simulink model "LADRC_24aV3_0"  (R2025a)
settings: Solver=VariableStepAuto  StartTime=0  StopTime=10  FixedStep=0.001  RelTol=1e-5
model workspace (MAT data in the model file):
  Amp = 0.0011
  P = 0
values from neighbouring files (symbols this model uses):
  A1 = 3.1416e-04    (= 0.00031416)    [InitialParameter.m]    (also in pneumatic_code.m = 0.000314159265359)
  A2 = 2.6389e-04    (= 0.00026389)    [InitialParameter.m]    (also in pneumatic_code.m = 0.000263893782902)
  Ar = 0.00005026    (= 5.026e-05)    [InitialParameter.m]    (also in pneumatic_code.m = 5.02654824574e-05)
  b = 1    [InitialParameter.m]    (also in pneumatic_code.m = 0.0025)
  beta = 50    [InitialParameter.m]
  bs = 0.008    [InitialParameter.m]
  ep = 0.0024    [InitialParameter.m]    (also in pneumatic_code.m = 0.02)
  g1 = 9    [InitialParameter.m]    (also in pneumatic_code.m = 10)
  g2 = 4    [InitialParameter.m]    (also in pneumatic_code.m = 9)
  g3 = 18    [InitialParameter.m]    (also in pneumatic_code.m = 5)
  g4 = 0.32    [InitialParameter.m]    (also in pneumatic_code.m = 3)
  g5 = 3    [pneumatic_code.m]
  k1 = wc^4    (= 81450625)    [InitialParameter.m]    (also in pneumatic_code.m = 3620506.28125)
  k2 = 4*wc^3    (= 3429500)    [InitialParameter.m]    (also in pneumatic_code.m = 883050.3125)
  k3 = 6*wc^2    (= 54150)    [InitialParameter.m]    (also in pneumatic_code.m = 86151.25)
  k4 = 4*wc    (= 380)    [InitialParameter.m]    (also in pneumatic_code.m = 4202.5)
  k5 = 5*(wc)    (= 102.5)    [pneumatic_code.m]
  Ke = 50    [InitialParameter.m]
  L = 0.15    [InitialParameter.m]    (also in pneumatic_code.m)
  M = 0.1    [InitialParameter.m]    (also in pneumatic_code.m)
  Ms = 0.5    [InitialParameter.m]    (also in pneumatic_code.m)
  Pa = 101352    [InitialParameter.m]
  Rs = 13.5    [InitialParameter.m]    (also in pneumatic_code.m)
  Vinact = 1e-04    (= 0.0001)    [InitialParameter.m]    (also in pneumatic_code.m)
  wall_force = 1e12    (= 1000000000000)    [InitialParameter.m]
  WallPos = 0.1    [InitialParameter.m]
undefined symbols (not defined in the file or in its folder): sigbuilder_block
libraries: slpidlib x1, SignalEditorBlockLib x1
settings Model: Creator=ply  LastModifiedBy=pangl
settings SolverCC: ZeroCrossAlgorithm=Adaptive
settings OptimizationCC: ZeroExternalMemoryAtStartup=off  ZeroInternalMemoryAtStartup=off
settings DebuggingCC: IgnoredZcDiagnostic=none  UnderSpecifiedDimensionMsg=warning
settings RTWCC: TargetLang=C++
settings GRTTargetCC: TargetLangStandard=C++11 (ISO)  CodeInterfacePackaging=C++ class

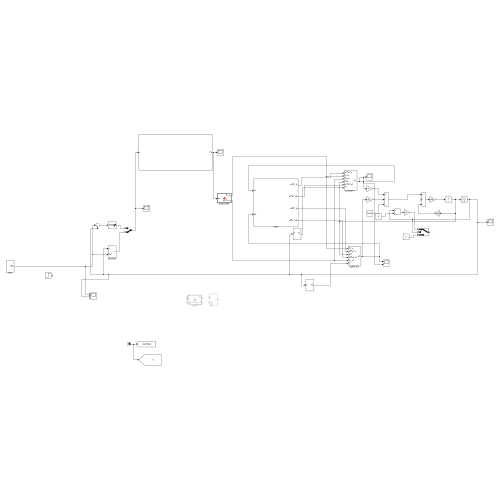
[thumbnail: Simulink's stored preview of the top-level diagram]
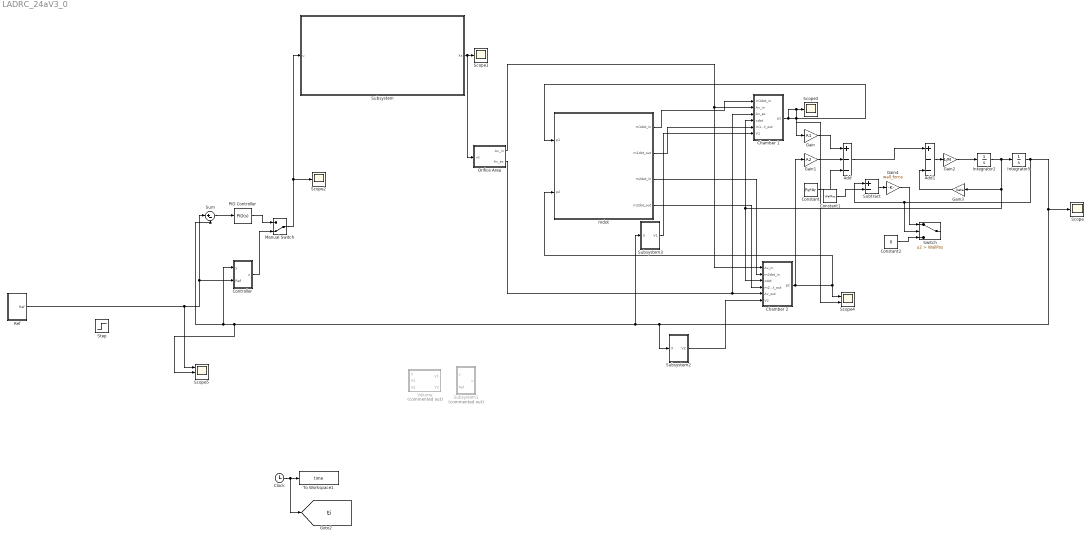
== system LADRC_24aV3_0 ==
  Add : Sum  Inputs=+--
  Add1 : Sum  Inputs=+--
  "Chamber 1 " : Subsystem
  Chamber 2 : Subsystem
  Clock : Clock
  Constant : Constant  Value=Pa*Ar
  Constant1 : Constant  Value=WallPos
  Constant2 : Constant  Value=0
  Controller : Subsystem
  Gain : Gain  Gain=A1
  Gain1 : Gain  Gain=A2
  Gain2 : Gain  Gain=1/M
  Gain3 : Gain  Gain=beta
  Gain4 : Gain  Gain=wall_force
  Integrator2 : Integrator
  Integrator5 : Integrator  InitialCondition=1e-4  LimitOutput=on  UpperSaturationLimit=0.15  LowerSaturationLimit=1e-4
  Manual Switch : ManualSwitch  CurrentSetting=0
  Orifice Area : MATLAB Function  TreatAsAtomicUnit=on
  PID Controller : slpidlib/PID Controller  Controller=PID  Form=Parallel  TimeDomain=Continuous-time  UseExternalTs=off  SampleTime=-1  IntegratorMethod=Forward Euler  FilterMethod=Forward Euler  ControllerParametersSource=internal  P=3800  I=420  UseKiTs=off  D=260  UseExternalDerivativeSource=off  N=4500  UseFilter=on  TunerSelectOption=Transfer Function Based (PID Tuner App)  InitialConditionSource=internal  InitialConditionForIntegrator=0  InitialConditionForFilter=19  DifferentiatorICPrevScaledInput=0  ExternalReset=none  TrackingMode=off  Kt=1  LimitOutput=on  SatLimitsSource=internal  UpperSaturationLimit=20  LowerSaturationLimit=-20  LinearizeAsGain=off  AntiWindupMode=clamping  Kb=2  LimitIntegrator=off  UpperIntegratorSaturationLimit=inf  LowerIntegratorSaturationLimit=-inf  POutMin=[]  POutMax=[]  IOutMin=[]  IOutMax=[]  DOutMin=[]  DOutMax=[]  NOutMin=[]  NOutMax=[]  SumOutMin=[]  SumOutMax=[]  SaturationOutMin=[]  SaturationOutMax=[]  PParamMin=[]  PParamMax=[]  IParamMin=[]  IParamMax=[]  DParamMin=[]  DParamMax=[]  NParamMin=[]  NParamMax=[]  KbParamMin=[]  KbParamMax=[]  KtParamMin=[]  KtParamMax=[]  KbOutMin=[]  KbOutMax=[]  KtOutMin=[]  KtOutMax=[]  IntegratorOutMin=[]  IntegratorOutMax=[]  FilterOutMin=[]  FilterOutMax=[]  SumI1OutMin=[]  SumI1OutMax=[]  SumI2OutMin=[]  SumI2OutMax=[]  SumI3OutMin=[]  SumI3OutMax=[]  SumI4OutMin=[]  SumI4OutMax=[]  SumDOutMin=[]  SumDOutMax=[]  DifferentiatorOutMin=[]  DifferentiatorOutMax=[]  FilterDiffOutCoefMin=[]  FilterDiffOutCoefMax=[]  ReciprocalOutMin=[]  ReciprocalOutMax=[]  SumDenOutMin=[]  SumDenOutMax=[]  SumNumOutMin=[]  SumNumOutMax=[]  DivideOutMin=[]  DivideOutMax=[]  UdiffTsProdOutMin=[]  UdiffTsProdOutMax=[]  NTsProdOutMin=[]  NTsProdOutMax=[]  UintegralTsProdOutMin=[]  UintegralTsProdOutMax=[]  UngainTsProdOutMin=[]  UngainTsProdOutMax=[]  ClampingZeroOutDataTypeStr=Inherit: Inherit via back propagation  ClampingZeroOutMin=[]  ClampingZeroOutMax=[]  FilterDenConstantOutDataTypeStr=Inherit: Inherit via back propagation  FilterDenConstantOutMin=[]  FilterDenConstantOutMax=[]  PCopyOutDataTypeStr=Inherit: Inherit via back propagation  PCopyOutMin=[]  PCopyOutMax=[]  NCopyOutDataTypeStr=Inherit: Inherit via back propagation  NCopyOutMin=[]  NCopyOutMax=[]  IntegratorContinuousStateAttributes=''  IntegratorStateMustResolveToSignalObject=off  IntegratorRTWStateStorageClass=Auto  FilterContinuousStateAttributes=''  FilterStateMustResolveToSignalObject=off  FilterRTWStateStorageClass=Auto  ParallelPVariant=InternalParameters  IdealPVariant=Disabled  IVariant=InternalParameters  DVariant=InternalParameters  IntegratorVariant=Continuous  SatVariant=Enabled  AWVariant=ContClampingParallel  PCopyVariant=Disabled  TRVariant=Disabled  FdbkBlocksVariant=Forward  IdealPFdbkVariant=Disabled  SatFdbkVariant=Disabled  DerivativeFilterVariant=ContFilter  NVariant=InternalParameters  NCopyVariant=Disabled  FilterICVariant=InternalICsFilter  IntegratorICVariant=InternalICs  ExternalResetVariant=Disabled  TRSumVariant=Passthrough  SumFdbkVariant=Disabled  SumVariant=Sum_PID  TsampFilterVariant=InternalTs  TsampNgainVariant=Passthrough  TsampIntegralVariant=Disabled_SignalSpec  ExternalSaturationOutDataTypeStr=Inherit: Same as second input  DerivativeSourceVariant=ErrorSignal  PreIntVariant=InternalPreInt
  Ref : Subsystem
  Scope{,1..3} (4 alike) : Scope
      Scope settings: ActiveDisplayYMinimum=-0.01125  ActiveDisplayYMaximum=0.10227
      Scope1 settings: ActiveDisplayYMinimum=-0.00138  ActiveDisplayYMaximum=0.00138  DataLoggingVariableName=ScopeData2
      Scope2 settings: ActiveDisplayYMinimum=-25  ActiveDisplayYMaximum=25  DataLoggingVariableName=ScopeData2
      Scope3 settings: ActiveDisplayYMinimum=39461.93859  ActiveDisplayYMaximum=658362.55266  DataLoggingVariableName=ScopeData3
  Scope4 : Scope  NumInputPorts=2
      settings: ActiveDisplayYMinimum=-74914.57533  ActiveDisplayYMaximum=775581.17798  DataLoggingVariableName=ScopeData4
  Scope5 : Scope  NumInputPorts=3
      settings: ActiveDisplayYMinimum=-0.030987006812028317  ActiveDisplayYMaximum=0.12320031519133484  DataLoggingVariableName=ScopeData7
  Step : Step  After=0.09  SampleTime=0
  Subsystem : Subsystem
  Subsystem1 : Subsystem  Commented=on
  Subsystem2 : Subsystem
  Subsystem3 : Subsystem
  Subtract : Sum  Inputs=+-
  Sum : Sum  Inputs=|+-
  Switch : Switch  Criteria=u2 > Threshold  Threshold=WallPos  SaturateOnIntegerOverflow=off  InputSameDT=off
  To Workspace1 : ToWorkspace  VariableName=time  SampleTime=-1
  Volume : MATLAB Function  Commented=on  TreatAsAtomicUnit=on
  mdot : Subsystem
  tag scope: ti=global
  wires:
  Integrator2/1 -> Gain3/1, Chamber 2/3(xdot), "Chamber 1 "/4(xdot), Integrator5/1
  "Chamber 1 "/1(p1) -> mdot/1(p1), Gain/1, Scope4/2, Scope3/1
  Orifice Area/1(Av_in) -> Chamber 2/1(Av_in), "Chamber 1 "/2(Av_in)
  Orifice Area/2(Av_ex) -> "Chamber 1 "/3(Av_ex), Chamber 2/5(Av_out)
  Chamber 2/1(p2) -> Scope4/1, mdot/2(p2), Gain1/1
  Subsystem/1(Xs) -> Orifice Area/1(xs), Scope1/1
  mdot/1(m1dot_in) -> "Chamber 1 "/1(m1dot_in)
  mdot/2(m1dot_out) -> "Chamber 1 "/5(m1dot_out)
  mdot/3(m2dot_in) -> Chamber 2/2(m2dot_in)
  mdot/4(m2dot_out) -> Chamber 2/4(m2dot_out)
  Integrator5/1 -> Switch/2, Subtract/1, Scope/1, Subsystem2/1(X), Subsystem3/1(X), Sum/2, Controller/1(y), Scope5/2
  Gain/1 -> Add/1
  Gain1/1 -> Add/2
  Constant/1 -> Add/3
  Add/1 -> Add1/1
  Gain3/1 -> Add1/3
  Add1/1 -> Gain2/1
  Constant1/1 -> Subtract/2
  Subtract/1 -> Gain4/1
  Gain4/1 -> Switch/1
  Constant2/1 -> Switch/3
  Subsystem3/1(V1) -> "Chamber 1 "/6(V1)
  Subsystem2/1(V2) -> Chamber 2/6(V2)
  Gain2/1 -> Integrator2/1
  Clock/1 -> [ti], To Workspace1/1
  PID Controller/1 -> Manual Switch/1
  Sum/1 -> PID Controller/1
  Controller/1(u) -> Manual Switch/2
  Manual Switch/1 -> Scope2/1, Subsystem/1(u)
  Ref/1(Ref) -> Sum/1, Controller/2(Ref), Scope5/1

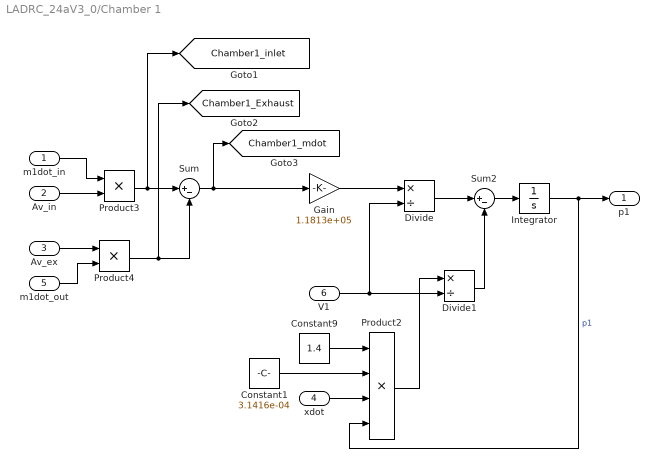
== system LADRC_24aV3_0/Chamber 1  ==
  m1dot_in : Inport
  Av_in : Inport  Port=2
  Av_ex : Inport  Port=3
  xdot : Inport  Port=4
  m1dot_out : Inport  Port=5
  V1 : Inport  Port=6
  Constant1 : Constant  Value=3.1416e-04
  Constant9 : Constant  Value=1.4
  Divide : Product  Inputs=*/
  Divide1 : Product  Inputs=*/
  Gain : Gain  Gain=1.1813e+05
  Integrator : Integrator  InitialCondition=101352  LimitOutput=on  UpperSaturationLimit=758423  LowerSaturationLimit=101352
  Product2 : Product  Inputs=4
  Product3 : Product
  Product4 : Product
  Sum : Sum  Inputs=|+-
  Sum2 : Sum  Inputs=|+-
  p1 : Outport
  tag scope: Chamber1_Exhaust=global, Chamber1_inlet=global, Chamber1_mdot=global
  wires:
  Divide/1 -> Sum2/1
  Sum/1 -> [Chamber1_mdot], Gain/1
  Gain/1 -> Divide/1
  Divide1/1 -> Sum2/2
  Constant9/1 -> Product2/1
  Product2/1 -> Divide1/1
  Integrator/1 -> p1/1, Product2/4  "p1"
  Sum2/1 -> Integrator/1
  m1dot_in/1 -> Product3/1
  xdot/1 -> Product2/3
  Product4/1 -> [Chamber1_Exhaust], Sum/2
  Av_in/1 -> Product3/2
  Product3/1 -> [Chamber1_inlet], Sum/1
  m1dot_out/1 -> Product4/2
  Av_ex/1 -> Product4/1
  Constant1/1 -> Product2/2
  V1/1 -> Divide/2, Divide1/2

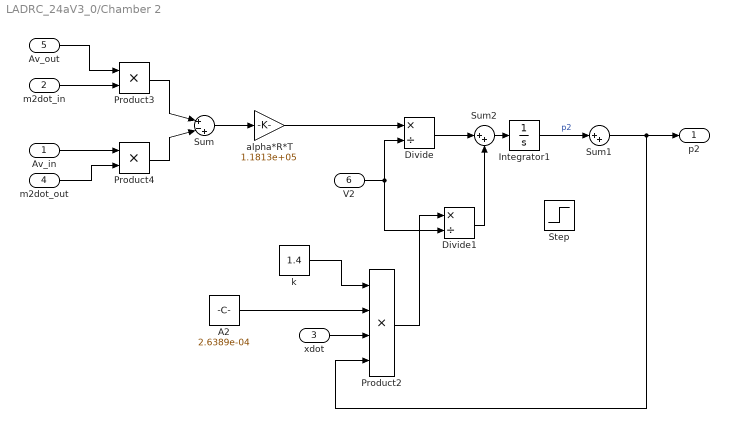
== system LADRC_24aV3_0/Chamber 2 ==
  Av_in : Inport
  m2dot_in : Inport  Port=2
  xdot : Inport  Port=3
  m2dot_out : Inport  Port=4
  Av_out : Inport  Port=5
  V2 : Inport  Port=6
  A2 : Constant  Value=2.6389e-04
  Divide : Product  Inputs=*/
  Divide1 : Product  Inputs=*/
  Integrator1 : Integrator  InitialCondition=10135  UpperSaturationLimit=75842  LowerSaturationLimit=10135
  Product2 : Product  Inputs=4
  Product3 : Product
  Product4 : Product
  Step : Step  Time=5  After=-10*10^3  SampleTime=0
  Sum : Sum  Inputs=|+-+
  Sum1 : Sum  Inputs=|++
  Sum2 : Sum  Inputs=|++
  alpha*R*T : Gain  Gain=1.1813e+05
  k : Constant  Value=1.4
  p2 : Outport
  wires:
  m2dot_out/1 -> Product4/2
  xdot/1 -> Product2/3
  Sum2/1 -> Integrator1/1
  Product2/1 -> Divide1/1
  k/1 -> Product2/1
  Divide1/1 -> Sum2/2
  A2/1 -> Product2/2
  alpha*R*T/1 -> Divide/1
  Sum/1 -> alpha*R*T/1
  Divide/1 -> Sum2/1
  Av_in/1 -> Product4/1
  m2dot_in/1 -> Product3/2
  Product3/1 -> Sum/1
  Av_out/1 -> Product3/1
  Product4/1 -> Sum/2
  V2/1 -> Divide/2, Divide1/2
  Integrator1/1 -> Sum1/1  "p2"
  Sum1/1 -> Product2/4, p2/1

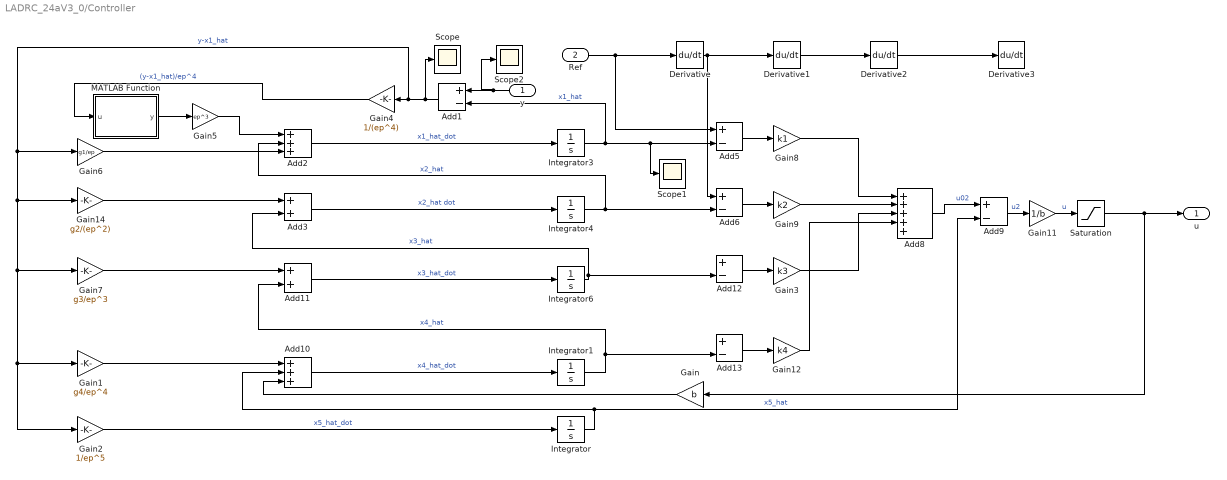
== system LADRC_24aV3_0/Controller ==
  y : Inport
  Ref : Inport  Port=2
  Add{1,5..6,9,12..13} (6 alike) : Sum  Inputs=+-
  Add10 : Sum  Inputs=+++
  Add11 : Sum
  Add2 : Sum  Inputs=+++
  Add3 : Sum
  Add8 : Sum  Inputs=+++++
  Derivative{,1..3} (4 alike) : Derivative
  Gain : Gain  Gain=b
  Gain1 : Gain  Gain=g4/ep^4
  Gain11 : Gain  Gain=1/b
  Gain12 : Gain  Gain=k4
  Gain14 : Gain  Gain=g2/(ep^2)
  Gain2 : Gain  Gain=1/ep^5
  Gain3 : Gain  Gain=k3
  Gain4 : Gain  Gain=1/(ep^4)
  Gain5 : Gain  Gain=ep^3
  Gain6 : Gain  Gain=g1/ep
  Gain7 : Gain  Gain=g3/ep^3
  Gain8 : Gain  Gain=k1
  Gain9 : Gain  Gain=k2
  Integrator{,1,4,6} (4 alike) : Integrator
  Integrator3 : Integrator  LimitOutput=on  UpperSaturationLimit=0.15  LowerSaturationLimit=1e-4
  MATLAB Function : MATLAB Function  TreatAsAtomicUnit=on
  Saturation : Saturate  UpperLimit=20  LowerLimit=-20
  Scope : Scope
      settings: ActiveDisplayYMinimum=-5.1E-5  ActiveDisplayYMaximum=4.9E-5
  Scope1 : Scope
      settings: ActiveDisplayYMinimum=-0.01864  ActiveDisplayYMaximum=0.16874  DataLoggingVariableName=ScopeData5
  Scope2 : Scope
      settings: ActiveDisplayYMinimum=-0.01149609845874263  ActiveDisplayYMaximum=0.10446488612868368  DataLoggingVariableName=ScopeData6
  u : Outport
  wires:
  Add12/1 -> Gain3/1
  Add6/1 -> Gain9/1
  Integrator3/1 -> Add1/2, Scope1/1, Add5/2  "x1_hat"
  Integrator4/1 -> Add2/2, Add6/2  "x2_hat"
  Integrator1/1 -> Add13/2, Add11/2  "x4_hat"
  Add13/1 -> Gain12/1
  Gain1/1 -> Add10/1
  Integrator/1 -> Add9/2, Add10/2  "x5_hat"
  Gain/1 -> Add10/3
  Gain7/1 -> Add11/1
  Gain5/1 -> Add2/1
  Gain11/1 -> Saturation/1  "u"
  Gain14/1 -> Add3/1
  Add11/1 -> Integrator6/1  "x3_hat_dot"
  Ref/1 -> Derivative/1, Add5/1
  Add1/1 -> Scope/1, Gain6/1, Gain2/1, Gain1/1, Gain7/1, Gain14/1, Gain4/1  "y-x1_hat"
  Gain6/1 -> Add2/3
  Add5/1 -> Gain8/1
  MATLAB Function/1(y) -> Gain5/1
  Integrator6/1 -> Add12/2, Add3/2  "x3_hat"
  Add9/1 -> Gain11/1  "u2"
  Add3/1 -> Integrator4/1  "x2_hat dot"
  Add2/1 -> Integrator3/1  "x1_hat_dot"
  y/1 -> Scope2/1, Add1/1
  Gain4/1 -> MATLAB Function/1(u)  "(y-x1_hat)/ep^4"
  Add10/1 -> Integrator1/1  "x4_hat_dot"
  Gain2/1 -> Integrator/1  "x5_hat_dot"
  Add8/1 -> Add9/1  "u02"
  Saturation/1 -> Gain/1, u/1
  Gain8/1 -> Add8/1
  Gain9/1 -> Add8/2
  Gain3/1 -> Add8/3
  Gain12/1 -> Add8/4
  Derivative/1 -> Add6/1, Derivative1/1
  Derivative1/1 -> Derivative2/1
  Derivative2/1 -> Derivative3/1

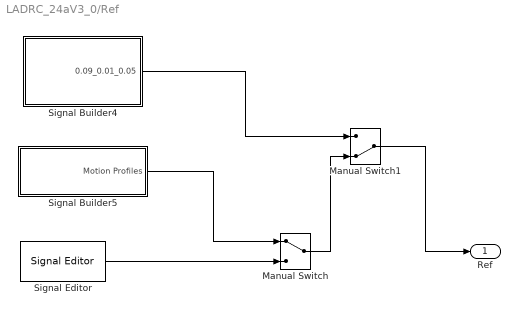
== system LADRC_24aV3_0/Ref ==
  Manual Switch : ManualSwitch
  Manual Switch1 : ManualSwitch  CurrentSetting=0
  Signal Builder4 : Subsystem  Tag=STV Subsys  LoadFcn=sigbuilder_block('load');  StartFcn=sigbuilder_block('start');  StopFcn=sigbuilder_block('stop');  ClipboardFcn=sigbuilder_block('clipboard');  mask(Sigbuilder block){tuvar=[0:10]}
      mask help: Simulink:masks:SigbuilderBlock_MD
      mask init:
      | if ~strcmp(get_param(bdroot(gcbh),'SimulationStatus'),'stopped') tuvar = sigbuilder_block('maskInit'); end
      settings: CopyFcn=sigbuilder_block('copy');  DeleteFcn=sigbuilder_block('delete');  ModelCloseFcn=sigbuilder_block('modelClose');  PreSaveFcn=sigbuilder_block('preSave');  PauseFcn=sigbuilder_block('pause');  ContinueFcn=sigbuilder_block('continue');  NameChangeFcn=sigbuilder_block('namechange');  OpenFcn=sigbuilder_block('open',[436.5 297.75 1045.5 630 ]);  CloseFcn=sigbuilder_block('close');
      mask Display: plot(0, 0, 100, 100,[2, 2, 32, 32, 2], [68, 8, 8, 68, 68],[32, 2], [38, 38], [32, 19, 2],[53, 60, 44], [32, 17, 17, 2],[16, 16, 31, 31]);txt = getActiveGroup(gcbh);text(2, 100, txt,'verticalAlignment', 'top');
  Signal Builder5 : Subsystem  Tag=STV Subsys  LoadFcn=sigbuilder_block('load');  StartFcn=sigbuilder_block('start');  StopFcn=sigbuilder_block('stop');  ClipboardFcn=sigbuilder_block('clipboard');  mask(Sigbuilder block){tuvar=[0:10]}
      mask help: Simulink:masks:SigbuilderBlock_MD
      mask init:
      | if ~strcmp(get_param(bdroot(gcbh),'SimulationStatus'),'stopped') tuvar = sigbuilder_block('maskInit'); end
      settings: CopyFcn=sigbuilder_block('copy');  DeleteFcn=sigbuilder_block('delete');  ModelCloseFcn=sigbuilder_block('modelClose');  PreSaveFcn=sigbuilder_block('preSave');  PauseFcn=sigbuilder_block('pause');  ContinueFcn=sigbuilder_block('continue');  NameChangeFcn=sigbuilder_block('namechange');  OpenFcn=sigbuilder_block('open',[5.4 84 1141.2 548 ]);  CloseFcn=sigbuilder_block('close');
      mask Display: plot(0, 0, 100, 100,[2, 2, 32, 32, 2], [68, 8, 8, 68, 68],[32, 2], [38, 38], [32, 19, 2],[53, 60, 44], [32, 17, 17, 2],[16, 16, 31, 31]);txt = getActiveGroup(gcbh);text(2, 100, txt,'verticalAlignment', 'top');
  Signal Editor : SignalEditorBlockLib/Signal Editor  FileName=ref_signal1.mat  ActiveScenario=Scenario  ActiveSignal=Pulse  IsBus=off  OutputBusObjectStr=Bus: BusObject  SampleTime=0  Interpolate=off  ZeroCross=off  OutputAfterFinalValue=Setting to zero  Unit=inherit  PreserveSignalName=on  ApplySigPropsToAllScenarios=on  ApplySigPropsToAllSignals=off  SignalPropertySource=Dialog parameters
  Ref : Outport
  wires:
  Signal Editor/1 -> Manual Switch/2
  Signal Builder5/1(Motion Profiles) -> Manual Switch/1
  Manual Switch/1 -> Manual Switch1/2
  Signal Builder4/1(0.09_0.01_0.05) -> Manual Switch1/1
  Manual Switch1/1 -> Ref/1

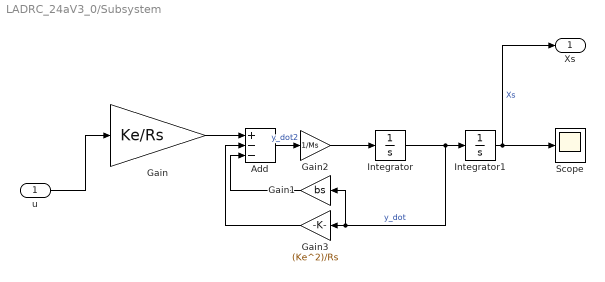
== system LADRC_24aV3_0/Subsystem ==
  u : Inport
  Add : Sum  Inputs=+--
  Gain : Gain  Gain=Ke/Rs
  Gain1 : Gain  Gain=bs
  Gain2 : Gain  Gain=1/Ms
  Gain3 : Gain  Gain=(Ke^2)/Rs
  Integrator : Integrator
  Integrator1 : Integrator  LimitOutput=on  UpperSaturationLimit=0.0011  LowerSaturationLimit=-0.0011
  Scope : Scope
      settings: ActiveDisplayYMinimum=-0.00138  ActiveDisplayYMaximum=0.00138
  Xs : Outport
  wires:
  Gain3/1 -> Add/2
  Gain/1 -> Add/1
  Add/1 -> Gain2/1  "y_dot2"
  Integrator1/1 -> Scope/1, Xs/1  "Xs"
  Integrator/1 -> Gain1/1, Gain3/1, Integrator1/1  "y_dot"
  u/1 -> Gain/1
  Gain1/1 -> Add/3
  Gain2/1 -> Integrator/1

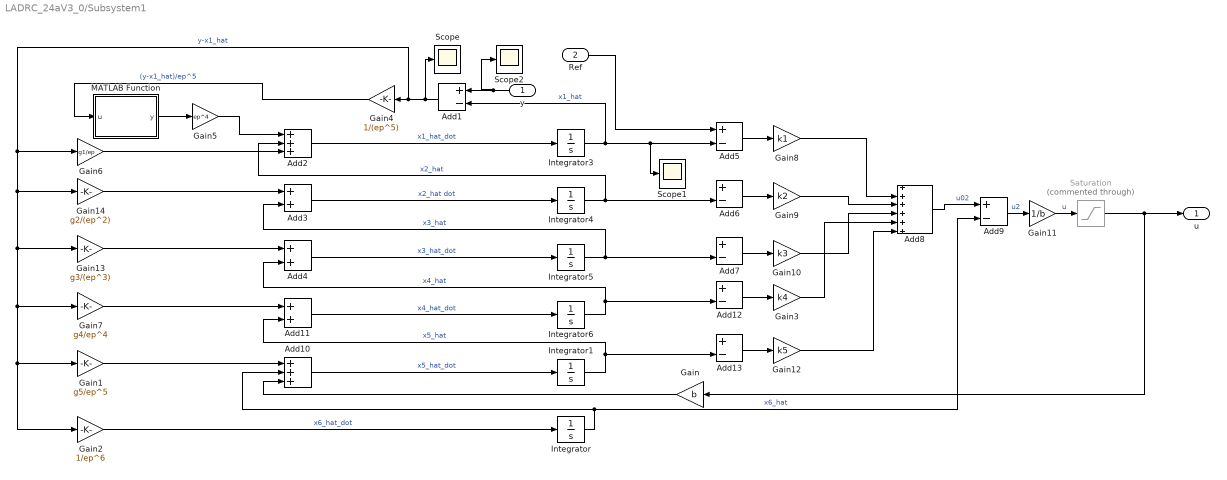
== system LADRC_24aV3_0/Subsystem1 ==
  y : Inport
  Ref : Inport  Port=2
  Add{1,5..7,9,12..13} (7 alike) : Sum  Inputs=+-
  Add10 : Sum  Inputs=+++
  Add11 : Sum
  Add2 : Sum  Inputs=+++
  Add3 : Sum
  Add4 : Sum
  Add8 : Sum  Inputs=++++++
  Gain : Gain  Gain=b
  Gain1 : Gain  Gain=g5/ep^5
  Gain10 : Gain  Gain=k3
  Gain11 : Gain  Gain=1/b
  Gain12 : Gain  Gain=k5
  Gain13 : Gain  Gain=g3/(ep^3)
  Gain14 : Gain  Gain=g2/(ep^2)
  Gain2 : Gain  Gain=1/ep^6
  Gain3 : Gain  Gain=k4
  Gain4 : Gain  Gain=1/(ep^5)
  Gain5 : Gain  Gain=ep^4
  Gain6 : Gain  Gain=g1/ep
  Gain7 : Gain  Gain=g4/ep^4
  Gain8 : Gain  Gain=k1
  Gain9 : Gain  Gain=k2
  Integrator{,1,4..6} (5 alike) : Integrator
  Integrator3 : Integrator  UpperSaturationLimit=0.15  LowerSaturationLimit=1e-4
  MATLAB Function : MATLAB Function  TreatAsAtomicUnit=on
  Saturation : Saturate  Commented=through  UpperLimit=5  LowerLimit=0
  Scope : Scope
      settings: ActiveDisplayYMinimum=-0.00018  ActiveDisplayYMaximum=0.00028
  Scope1 : Scope
      settings: ActiveDisplayYMinimum=-0.01864  ActiveDisplayYMaximum=0.16874  DataLoggingVariableName=ScopeData5
  Scope2 : Scope
      settings: ActiveDisplayYMinimum=-0.01549  ActiveDisplayYMaximum=0.14038  DataLoggingVariableName=ScopeData6
  u : Outport
  wires:
  Add12/1 -> Gain3/1
  Add6/1 -> Gain9/1
  Integrator3/1 -> Add1/2, Scope1/1, Add5/2  "x1_hat"
  Integrator4/1 -> Add6/2, Add2/2  "x2_hat"
  Integrator1/1 -> Add13/2, Add11/2  "x5_hat"
  Gain12/1 -> Add8/6
  Add13/1 -> Gain12/1
  Gain1/1 -> Add10/1
  Integrator/1 -> Add9/2, Add10/2  "x6_hat"
  Gain/1 -> Add10/3
  Gain7/1 -> Add11/1
  Gain5/1 -> Add2/1
  Gain11/1 -> Saturation/1  "u"
  Gain14/1 -> Add3/1
  Add11/1 -> Integrator6/1  "x4_hat_dot"
  Ref/1 -> Add5/1
  Gain10/1 -> Add8/4
  Add4/1 -> Integrator5/1  "x3_hat_dot"
  Add1/1 -> Scope/1, Gain6/1, Gain2/1, Gain1/1, Gain7/1, Gain13/1, Gain14/1, Gain4/1  "y-x1_hat"
  Gain3/1 -> Add8/5
  Gain6/1 -> Add2/3
  Add5/1 -> Gain8/1
  Integrator5/1 -> Add7/2, Add3/2  "x3_hat"
  Add7/1 -> Gain10/1
  MATLAB Function/1(y) -> Gain5/1
  Integrator6/1 -> Add12/2, Add4/2  "x4_hat"
  Add9/1 -> Gain11/1  "u2"
  Gain8/1 -> Add8/2
  Add3/1 -> Integrator4/1  "x2_hat dot"
  Add2/1 -> Integrator3/1  "x1_hat_dot"
  y/1 -> Scope2/1, Add1/1
  Gain9/1 -> Add8/3
  Gain4/1 -> MATLAB Function/1(u)  "(y-x1_hat)/ep^5"
  Gain13/1 -> Add4/1
  Add10/1 -> Integrator1/1  "x5_hat_dot"
  Gain2/1 -> Integrator/1  "x6_hat_dot"
  Add8/1 -> Add9/1  "u02"
  Saturation/1 -> Gain/1, u/1

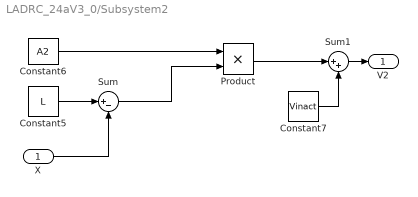
== system LADRC_24aV3_0/Subsystem2 ==
  X : Inport
  Constant5 : Constant  Value=L
  Constant6 : Constant  Value=A2
  Constant7 : Constant  Value=Vinact
  Product : Product
  Sum : Sum  Inputs=|+-
  Sum1 : Sum  Inputs=|++
  V2 : Outport
  wires:
  Constant7/1 -> Sum1/2
  X/1 -> Sum/2
  Constant5/1 -> Sum/1
  Product/1 -> Sum1/1
  Constant6/1 -> Product/1
  Sum1/1 -> V2/1
  Sum/1 -> Product/2

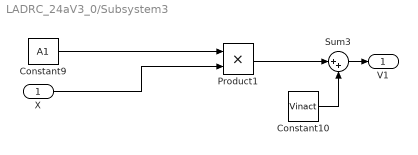
== system LADRC_24aV3_0/Subsystem3 ==
  X : Inport
  Constant10 : Constant  Value=Vinact
  Constant9 : Constant  Value=A1
  Product1 : Product
  Sum3 : Sum  Inputs=|++
  V1 : Outport
  wires:
  Constant10/1 -> Sum3/2
  Product1/1 -> Sum3/1
  Constant9/1 -> Product1/1
  X/1 -> Product1/2
  Sum3/1 -> V1/1

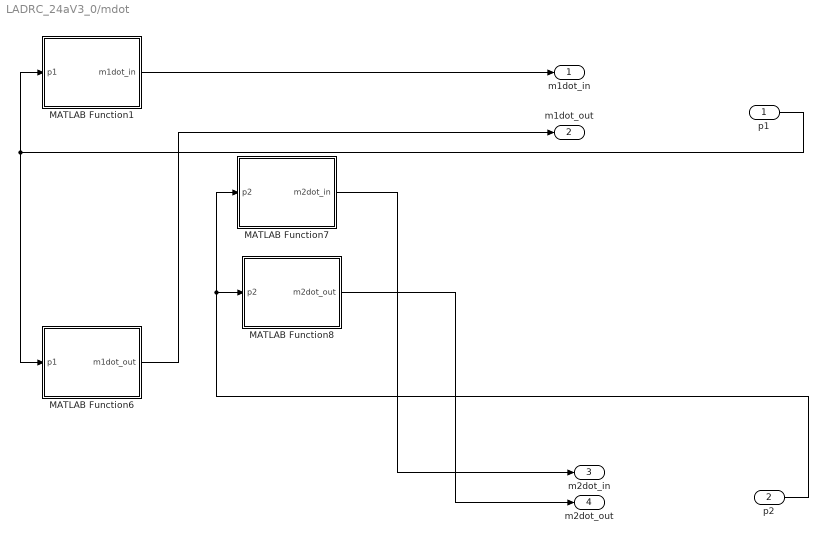
== system LADRC_24aV3_0/mdot ==
  p1 : Inport
  p2 : Inport  Port=2
  MATLAB Function1 : MATLAB Function  TreatAsAtomicUnit=on
  MATLAB Function6 : MATLAB Function  TreatAsAtomicUnit=on
  MATLAB Function7 : MATLAB Function  TreatAsAtomicUnit=on
  MATLAB Function8 : MATLAB Function  TreatAsAtomicUnit=on
  m1dot_in : Outport
  m1dot_out : Outport  Port=2
  m2dot_in : Outport  Port=3
  m2dot_out : Outport  Port=4
  wires:
  MATLAB Function7/1(m2dot_in) -> m2dot_in/1
  MATLAB Function6/1(m1dot_out) -> m1dot_out/1
  MATLAB Function1/1(m1dot_in) -> m1dot_in/1
  p1/1 -> MATLAB Function1/1(p1), MATLAB Function6/1(p1)
  MATLAB Function8/1(m2dot_out) -> m2dot_out/1
  p2/1 -> MATLAB Function7/1(p2), MATLAB Function8/1(p2)

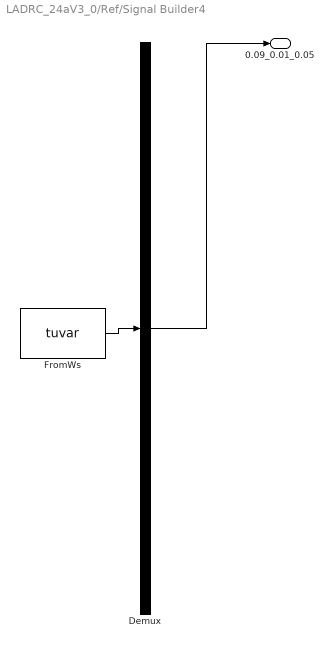
== system LADRC_24aV3_0/Ref/Signal Builder4 ==
  Demux : Demux  Tag=STV Demux  Outputs=1
      settings: DisplayOption=none
  FromWs : FromWorkspace  Tag=STV FromWs  VariableName=tuvar
      SigBuilderData=|
      | common.afterFinalStr = 'Extrapolate'
      | common.sampleTime = 0
      | dataSet.timeRange = [0 6]
      | dataSet.name = 'Group 1'
      | sbobj.Groups.Name = 'Group 1'
      | sbobj.Groups.Signals.Name = '0.09_0.01_0.05'
      | sbobj.Groups.Signals.XData = [0 2 2 4 4 6]
      | sbobj.Groups.Signals.YData = [0.09 0.09 0.01 0.01 0.05 0.05]
      | sbobj.Groups.TimeRange = [0 6]
  0.09_0.01_0.05 : Outport  Tag=STV Outport
  wires:
  Demux/1 -> 0.09_0.01_0.05/1
  FromWs/1 -> Demux/1

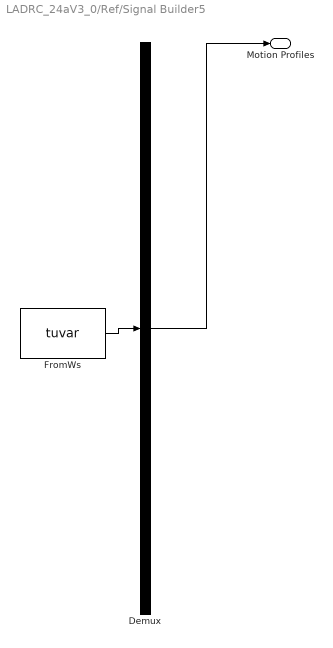
== system LADRC_24aV3_0/Ref/Signal Builder5 ==
  Demux : Demux  Tag=STV Demux  Outputs=1
      settings: DisplayOption=none
  FromWs : FromWorkspace  Tag=STV FromWs  VariableName=tuvar
      SigBuilderData=|
      | common.afterFinalStr = 'Extrapolate'
      | common.sampleTime = 0
      | dataSet.timeRange = [0 10]
      | dataSet.name = 'Group 1'
      | sbobj.Groups.Name = 'Group 1'
      | sbobj.Groups.Signals.Name = 'Motion Profiles'
      | sbobj.Groups.Signals.XData = [0 0.4 1 1.4 2 3.6 4 5.4 6 8 8.6 10]
      | sbobj.Groups.Signals.YData = [0.02 0.02 0.02 0.09 0.09 0.0898 0.02 0.02 0.06 0.06 0.0196 0.02]
  Motion Profiles : Outport  Tag=STV Outport
  wires:
  Demux/1 -> Motion Profiles/1
  FromWs/1 -> Demux/1

== matlab function LADRC_24aV3_0/mdot/MATLAB Function1 ==
  data: p1 input; m1dot_in output
% function [m_dot_in,m_dot_out] = massflowrate(Avin,Avout,Pd,Pu)
% % C1 = sqrt(k/R*(2/(k+1)^((k+1)/(k-1))));
% % C2 = sqrt(2*k/(R*(k-1)));
% %Pu = 758420;
% 
% C1 = 0.0404;
% C2 = 0.1561;
% Pcr = 0.528;
% Cf=0.25;
% k = 1.4;
% T = 294;
% if (Pd/Pu)<Pcr
%     m_dot_in = Cf*Avin*C1*Pu/sqrt(T);
%     m_dot_out = Cf*Avout*C1*Pu/sqrt(T);
% elseif (Pd/Pu)>Pcr
%     m_dot_in = Cf*Avin*C2*Pu/sqrt(T)*(Pd/Pu)^(1/k)*sqrt(1-((Pd/Pu)^((k-1)/k)));
%     m_dot_out = Cf*Avout*C2*Pu/sqrt(T)*(Pd/Pu)^(1/k)*sqrt(1-((Pd/Pu)^((k-1)/k)));
% else
%     m_dot_in = 0;
%     m_dot_out = 0;
% end
% 
% 
% end

function m1dot_in = fcn(p1)
C1 = 0.0404;
C2 = 0.1561;
Pcr = 0.528;
Cf=0.25;
k = 1.4;
T = 294;
Ps=758423;      %Source Pressure
Patm=101352;    %Atmosphereic pressure
if (p1<Patm)
    p1=Patm;
elseif (p1>Ps)
    p1=Ps;
end
pu=Ps;
pd=p1;
Pratio=pd/pu;
if(Pratio <= Pcr && Pratio > 0)
    m1dot_in = Cf*C1*pu/sqrt(T);
elseif (Pratio > Pcr)
    m1dot_in = Cf*C2*pu/sqrt(T)*(pd/pu)^(1/k)*sqrt(1-(pd/pu)^((k-1)/k));
else
    m1dot_in = 0;
end

== matlab function LADRC_24aV3_0/Orifice Area ==
  data: xs input; Av_in output; Av_ex output
function [Av_in,Av_ex] = fcn(xs)
Xs = abs(xs);
nh = 4;
Pw = 0.0024;
Rh = 0.0019;
if (xs <= (Pw-Rh))
    Av_in=0;
elseif (xs >= (Pw+Rh))
    Av_in=pi*nh*Rh^2;
else
    temp=sqrt((Rh-Pw+abs(xs))/(Rh+Pw-abs(xs)));
    Av_in=nh*((2*Rh*Rh*atan(temp))-((Pw-xs)*(sqrt((Rh^2)-(Pw-xs)^2))));
end

if (xs <= (-Pw-Rh))
    Av_ex=pi*nh*Rh^2;
elseif (xs >= (Rh-Pw))
    Av_ex=0;
else
    temp1=sqrt((Rh-Pw+Xs)/(Rh+Pw-Xs));
    Av_ex=nh*((2*Rh*Rh*atan(temp1))-((Pw-Xs)*(sqrt((Rh^2)-(Pw-Xs)^2))));
end
end

== matlab function LADRC_24aV3_0/Subsystem1/MATLAB Function ==
  data: u input; y output
function y = fcn(u)
y = 0;
if u <= -pi/2
    y = -(1/(4*pi));
elseif u <= pi/2 && u >= -pi/2
    y = sin(u)/(4*pi);
elseif u >=pi/2
    y = 1/(4*pi);
end

== matlab function LADRC_24aV3_0/Volume ==
  data: V1 output; V2 output; X input; A1 input; A2 input
function [V1,V2] = Volume(X,A1,A2)
V01 = 10e-4;
V02 = 10e-4;
L = 0.15;
V1 = V01+(A1*X);
V2 = V02+(A2*(L-X));

end

== matlab function LADRC_24aV3_0/Controller/MATLAB Function ==
  data: u input; y output
function y = fcn(u)
y = 0;
if u <= -pi/2
    y = -(1/(4*pi));
elseif u <= pi/2 && u >= -pi/2
    y = sin(u)/(4*pi);
elseif u >=pi/2
    y = 1/(4*pi);
end

== matlab function LADRC_24aV3_0/mdot/MATLAB Function6 ==
  data: p1 input; m1dot_out output
function m1dot_out = fcn(p1)
C1 = 0.0404;
C2 = 0.1561;
Pcr = 0.528;
Cf=0.25;
k = 1.4;
T = 294;
Ps=758423;      %Source Pressure
Patm=101352;    %Atmosphereic pressure
if (p1<Patm)
    p1=Patm;
elseif (p1>Ps)
    p1=Ps;
end
pu=p1;
pd=Patm;
Pratio=pd/pu;
if(Pratio <= Pcr && Pratio > 0)
    m1dot_out = Cf*C1*pu/sqrt(T);
elseif (Pratio > Pcr)
    m1dot_out = Cf*C2*pu/sqrt(T)*(pd/pu)^(1/k)*sqrt(1-(pd/pu)^((k-1)/k));
else
    m1dot_out = 0;
end

== matlab function LADRC_24aV3_0/mdot/MATLAB Function7 ==
  data: p2 input; m2dot_in output
function m2dot_in = fcn(p2)
C1 = 0.0404;
C2 = 0.1561;
Pcr = 0.528;
Cf=0.25;
k = 1.4;
T = 294;
Ps=758423;      %Source Pressure
Patm=101352;    %Atmosphereic pressure
if (p2<Patm)
    p2=Patm;
elseif (p2>Ps)
    p2=Ps;
end
pu=Ps;
pd=p2;
Pratio=pd/pu;
if(Pratio <= Pcr && Pratio > 0)
    m2dot_in = Cf*C1*pu/sqrt(T);
elseif (Pratio > Pcr)
    m2dot_in = Cf*C2*pu/sqrt(T)*(pd/pu)^(1/k)*sqrt(1-(pd/pu)^((k-1)/k));
else
    m2dot_in = 0;
end

== matlab function LADRC_24aV3_0/mdot/MATLAB Function8 ==
  data: p2 input; m2dot_out output
function m2dot_out = fcn(p2)
C1 = 0.0404;
C2 = 0.1561;
Pcr = 0.528;
Cf=0.25;
k = 1.4;
T = 294;
Ps=758423;      %Source Pressure
Patm=101352;    %Atmosphereic pressure
if (p2<Patm)
    p2=Patm;
elseif (p2>Ps)
    p2=Ps;
end
pu=p2;
pd=Patm;
Pratio=pd/pu;
if(Pratio <= Pcr && Pratio > 0)
    m2dot_out = Cf*C1*pu/sqrt(T);
elseif (Pratio > Pcr)
    m2dot_out = Cf*C2*pu/sqrt(T)*(pd/pu)^(1/k)*sqrt(1-(pd/pu)^((k-1)/k));
else
    m2dot_out = 0;
end
